simulink model "Simulink Deliverable 1"  (R2020a)
settings: Solver=FixedStepAuto  StartTime=0.0  StopTime=10.0  FixedStep=1e-3  RelTol=1e-3  EnableMultiTasking=on
undefined symbols (not defined in the file or in its folder): D0, D1, D10, D11, D12, D13, D2, D3, D4, D5, D6, D7, D8, D9, PTA0, PTA1, PTA2, PTB23, PTB9, PTC16, PTC17, PTC2, PTC3, PTC4, PTD0, PTD1, PTD2, PTD3
libraries: frdmk64flib x17
settings Model: ExtModeTrigDuration=5  Creator=shivr  LastModifiedBy=22538
settings OptimizationCC: EnhancedBackFolding=on  PassReuseOutputArgsAs=Individual arguments  ZeroExternalMemoryAtStartup=off  ZeroInternalMemoryAtStartup=off  MaxStackSize=64  OptimizeBlockOrder=speed  DifferentSizesBufferReuse=on  OptimizationCustomize=off  EfficientTunableParamExpr=on
settings DebuggingCC: ParameterTunabilityLossMsg=error
settings HardwareCC: ProdBitPerPointer=32  ProdBitPerSizeT=32  ProdBitPerPtrDiffT=32  ProdLargestAtomicInteger=Long  ProdLargestAtomicFloat=Double  ProdWordSize=32  ProdHWDeviceType=ARM Compatible->ARM Cortex
settings SFSimCC: MATLABDynamicMemAlloc=off
settings RTWCC: SystemTargetFile=ert.tlc  HardwareBoard=NXP FRDM-K64F  TemplateMakefile=ert_default_tmf  Toolchain=GNU Tools for ARM Embedded Processors
settings CodeAppCC: ForceParamTrailComments=on  IgnoreCustomStorageClasses=off  OperatorAnnotations=on  SimulinkDataObjDesc=on  SFDataObjDesc=on  InsertBlockDesc=on

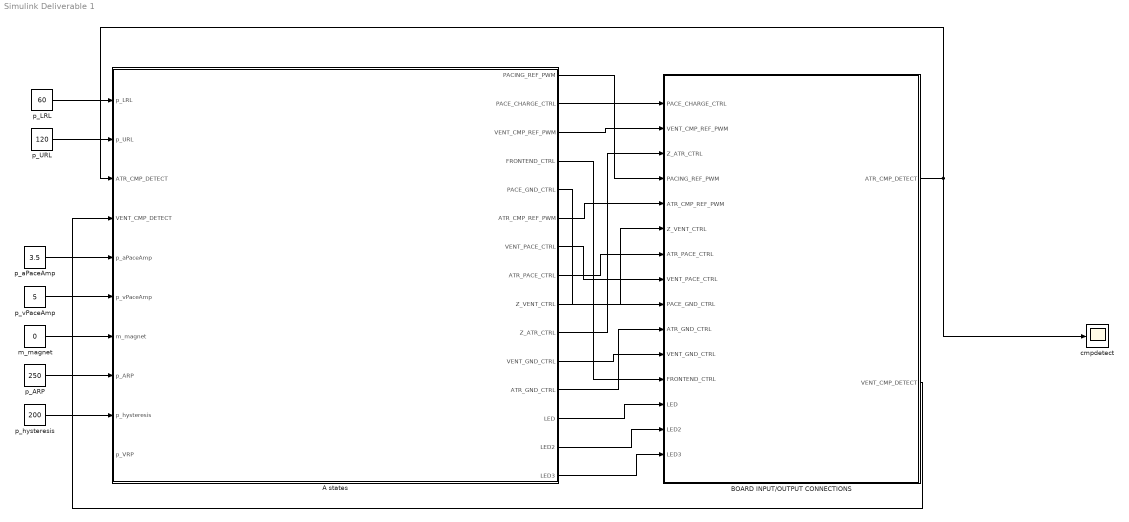
== system Simulink Deliverable 1 ==
  A states : Subsystem
  BOARD INPUT/OUTPUT CONNECTIONS : Subsystem
  cmpdetect : Scope
  m_magnet : Constant  Value=0
  p_ARP : Constant  Value=250
  p_LRL : Constant  Value=60
  p_URL : Constant  Value=120
  p_aPaceAmp : Constant  Value=3.5
  p_hysteresis : Constant  Value=200
  p_vPaceAmp : Constant  Value=5
  wires:
  p_LRL/1 -> A states/1(p_LRL)
  A states/12(ATR_GND_CTRL) -> BOARD INPUT/OUTPUT CONNECTIONS/10(ATR_GND_CTRL)
  A states/5(PACE_GND_CTRL) -> BOARD INPUT/OUTPUT CONNECTIONS/9(PACE_GND_CTRL)
  A states/11(VENT_GND_CTRL) -> BOARD INPUT/OUTPUT CONNECTIONS/11(VENT_GND_CTRL)
  A states/7(VENT_PACE_CTRL) -> BOARD INPUT/OUTPUT CONNECTIONS/8(VENT_PACE_CTRL)
  A states/8(ATR_PACE_CTRL) -> BOARD INPUT/OUTPUT CONNECTIONS/7(ATR_PACE_CTRL)
  A states/9(Z_VENT_CTRL) -> BOARD INPUT/OUTPUT CONNECTIONS/6(Z_VENT_CTRL)
  A states/10(Z_ATR_CTRL) -> BOARD INPUT/OUTPUT CONNECTIONS/3(Z_ATR_CTRL)
  A states/4(FRONTEND_CTRL) -> BOARD INPUT/OUTPUT CONNECTIONS/12(FRONTEND_CTRL)
  A states/2(PACE_CHARGE_CTRL) -> BOARD INPUT/OUTPUT CONNECTIONS/1(PACE_CHARGE_CTRL)
  A states/1(PACING_REF_PWM) -> BOARD INPUT/OUTPUT CONNECTIONS/4(PACING_REF_PWM)
  A states/13(LED) -> BOARD INPUT/OUTPUT CONNECTIONS/13(LED)
  p_URL/1 -> A states/2(p_URL)
  BOARD INPUT/OUTPUT CONNECTIONS/1(ATR_CMP_DETECT) -> A states/3(ATR_CMP_DETECT), cmpdetect/1
  BOARD INPUT/OUTPUT CONNECTIONS/2(VENT_CMP_DETECT) -> A states/4(VENT_CMP_DETECT)
  p_aPaceAmp/1 -> A states/5(p_aPaceAmp)
  m_magnet/1 -> A states/7(m_magnet)
  A states/14(LED2) -> BOARD INPUT/OUTPUT CONNECTIONS/14(LED2)
  p_vPaceAmp/1 -> A states/6(p_vPaceAmp)
  A states/6(ATR_CMP_REF_PWM) -> BOARD INPUT/OUTPUT CONNECTIONS/5(ATR_CMP_REF_PWM)
  p_ARP/1 -> A states/8(p_ARP)
  p_hysteresis/1 -> A states/9(p_hysteresis)
  A states/15(LED3) -> BOARD INPUT/OUTPUT CONNECTIONS/15(LED3)
  A states/3(VENT_CMP_REF_PWM) -> BOARD INPUT/OUTPUT CONNECTIONS/2(VENT_CMP_REF_PWM)

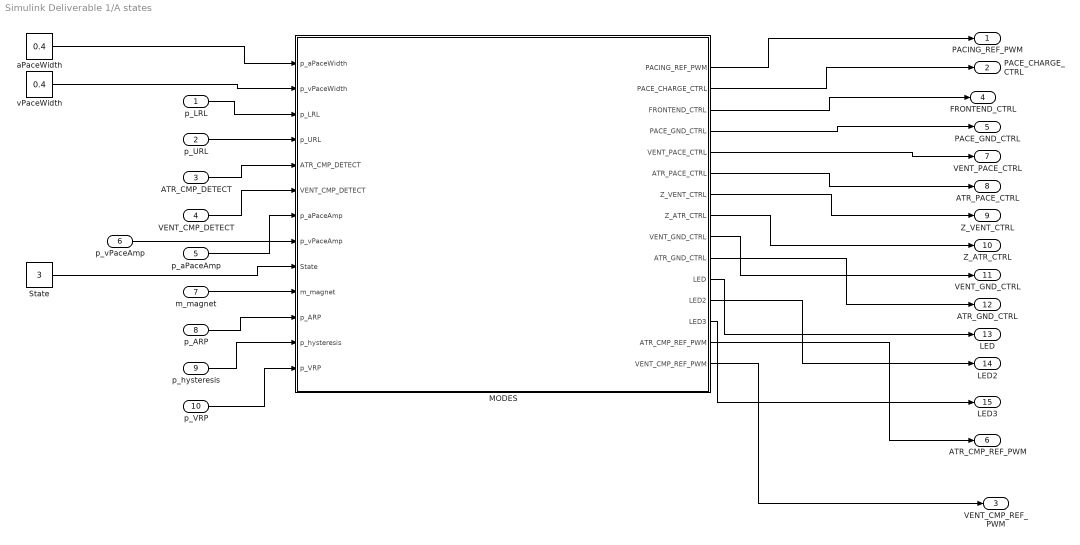
== system Simulink Deliverable 1/A states ==
  p_LRL : Inport
  p_URL : Inport  Port=2
  ATR_CMP_DETECT : Inport  Port=3
  VENT_CMP_DETECT : Inport  Port=4
  p_aPaceAmp : Inport  Port=5
  p_vPaceAmp : Inport  Port=6
  m_magnet : Inport  Port=7
  p_ARP : Inport  Port=8
  p_hysteresis : Inport  Port=9
  p_VRP : Inport  Port=10
  MODES : Stateflow chart  TreatAsAtomicUnit=on
      settings: PortSchema="{\"entries\":[{\"content\":{\"sides\":[{\"content\":{\"connectorIds\":[\"In1\",\"In2\",\"In3\",\"In4\",\"In5\",\"In6\",\"In7\",\"In8\",\"In9\",\"In10\",\"In11\",\"In12\",\"In13\"]},\"type\":\"ConnectorPlacement.EquallySpacedRectSide\",\"uuid\":\"8502a3c5-6307-4e02-81ee-17e1a35cc298\"},{\"content\":{\"connectorIds\":[\"Out1\",\"Out2\",\"Out3\",\"Out4\",\"Out5\",\"Out6\",\"Out7\",\"Out8\",\"Out9\",\"Out10\",\"Out11\",\"Out14\",\"Out13\",\"Out12\",\"Out15\"],\"side\":\"RIGHT\"},\"type\":\"ConnectorPlacement.EquallySpacedRectSide\",\"uuid\":\"71555ad9-e88e-4949-94fd-af1b739ca2ca\"},{\"content\":{\"connectorIds\":[],\"side\":\"TOP\"},\"type\":\"ConnectorPlacement.EquallySpacedRectSide\",\"uuid\":\"f0239cae-2fc2-4d44-ac00-93735ab3ef8c\"},{\"content\":{\"connectorIds\":[],\"side\":\"BOTTOM\"},\"type\":\"ConnectorPlacement.EquallySpacedRectSide\",\"uuid\":\"7d1612d5-a202-47d8-98e6-e2ca77499232\"}]},\"type\":\"ConnectorPlacement.EquallySpacedConnector\",\"uuid\":\"0a066545-78b2-4ddc-84c3-90461cea3699\"}],\"packageUris\":[\"http://schema.mathworks.com/mf0/Connector/19700101\"],\"version\":\"1.0\"}"
  State : Constant  Value=3
  aPaceWidth : Constant  Value=0.4
  vPaceWidth : Constant  Value=0.4
  PACING_REF_PWM : Outport
  PACE_CHARGE_CTRL : Outport  Port=2
  VENT_CMP_REF_PWM : Outport  Port=3
  FRONTEND_CTRL : Outport  Port=4
  PACE_GND_CTRL : Outport  Port=5
  ATR_CMP_REF_PWM : Outport  Port=6
  VENT_PACE_CTRL : Outport  Port=7
  ATR_PACE_CTRL : Outport  Port=8
  Z_VENT_CTRL : Outport  Port=9
  Z_ATR_CTRL : Outport  Port=10
  VENT_GND_CTRL : Outport  Port=11
  ATR_GND_CTRL : Outport  Port=12
  LED : Outport  Port=13
  LED2 : Outport  Port=14
  LED3 : Outport  Port=15
  wires:
  aPaceWidth/1 -> MODES/1(p_aPaceWidth)
  MODES/5(VENT_PACE_CTRL) -> VENT_PACE_CTRL/1
  MODES/3(FRONTEND_CTRL) -> FRONTEND_CTRL/1
  MODES/1(PACING_REF_PWM) -> PACING_REF_PWM/1
  MODES/6(ATR_PACE_CTRL) -> ATR_PACE_CTRL/1
  MODES/7(Z_VENT_CTRL) -> Z_VENT_CTRL/1
  MODES/4(PACE_GND_CTRL) -> PACE_GND_CTRL/1
  MODES/8(Z_ATR_CTRL) -> Z_ATR_CTRL/1
  MODES/2(PACE_CHARGE_CTRL) -> PACE_CHARGE_CTRL/1
  MODES/9(VENT_GND_CTRL) -> VENT_GND_CTRL/1
  MODES/10(ATR_GND_CTRL) -> ATR_GND_CTRL/1
  MODES/11(LED) -> LED/1
  p_LRL/1 -> MODES/3(p_LRL)
  p_URL/1 -> MODES/4(p_URL)
  ATR_CMP_DETECT/1 -> MODES/5(ATR_CMP_DETECT)
  VENT_CMP_DETECT/1 -> MODES/6(VENT_CMP_DETECT)
  p_aPaceAmp/1 -> MODES/7(p_aPaceAmp)
  State/1 -> MODES/9(State)
  m_magnet/1 -> MODES/10(m_magnet)
  MODES/14(LED2) -> LED2/1
  vPaceWidth/1 -> MODES/2(p_vPaceWidth)
  p_vPaceAmp/1 -> MODES/8(p_vPaceAmp)
  MODES/12(ATR_CMP_REF_PWM) -> ATR_CMP_REF_PWM/1
  p_ARP/1 -> MODES/11(p_ARP)
  p_hysteresis/1 -> MODES/12(p_hysteresis)
  MODES/13(LED3) -> LED3/1
  p_VRP/1 -> MODES/13(p_VRP)
  MODES/15(VENT_CMP_REF_PWM) -> VENT_CMP_REF_PWM/1

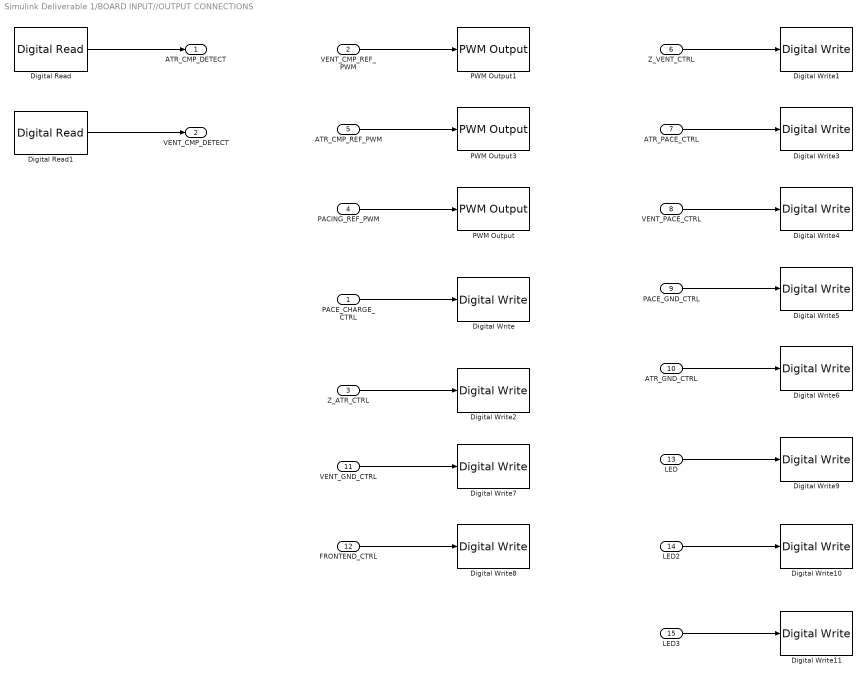
== system Simulink Deliverable 1/BOARD INPUT//OUTPUT CONNECTIONS ==
  PACE_CHARGE_CTRL : Inport
  VENT_CMP_REF_PWM : Inport  Port=2
  Z_ATR_CTRL : Inport  Port=3
  PACING_REF_PWM : Inport  Port=4
  ATR_CMP_REF_PWM : Inport  Port=5
  Z_VENT_CTRL : Inport  Port=6
  ATR_PACE_CTRL : Inport  Port=7
  VENT_PACE_CTRL : Inport  Port=8
  PACE_GND_CTRL : Inport  Port=9
  ATR_GND_CTRL : Inport  Port=10
  VENT_GND_CTRL : Inport  Port=11
  FRONTEND_CTRL : Inport  Port=12
  LED : Inport  Port=13
  LED2 : Inport  Port=14
  LED3 : Inport  Port=15
  Digital Read : frdmk64flib/Digital Read  Whichpin=PTC16 (D0)  SampleTime=-1
  Digital Read1 : frdmk64flib/Digital Read  Whichpin=PTC17 (D1)  SampleTime=-1
  Digital Write : frdmk64flib/Digital Write  Whichpin=PTB9 (D2)
  Digital Write1 : frdmk64flib/Digital Write  Whichpin=PTC3 (D7)
  Digital Write10 : frdmk64flib/Digital Write  Whichpin=BLUE_LED
  Digital Write11 : frdmk64flib/Digital Write  Whichpin=GREEN_LED
  Digital Write2 : frdmk64flib/Digital Write  Whichpin=PTB23 (D4)
  Digital Write3 : frdmk64flib/Digital Write  Whichpin=PTA0 (D8)
  Digital Write4 : frdmk64flib/Digital Write  Whichpin=PTC4 (D9)
  Digital Write5 : frdmk64flib/Digital Write  Whichpin=PTD0 (D10)
  Digital Write6 : frdmk64flib/Digital Write  Whichpin=PTD2 (D11)
  Digital Write7 : frdmk64flib/Digital Write  Whichpin=PTD3 (D12)
  Digital Write8 : frdmk64flib/Digital Write  Whichpin=PTD1 (D13)
  Digital Write9 : frdmk64flib/Digital Write  Whichpin=RED_LED
  PWM Output : frdmk64flib/PWM Output  Whichpin=PTA2 (D5)  InitialFrequency=2000  InitialDutyCycle=0
  PWM Output1 : frdmk64flib/PWM Output  Whichpin=PTA1 (D3)  InitialFrequency=2000  InitialDutyCycle=0
  PWM Output3 : frdmk64flib/PWM Output  Whichpin=PTC2 (D6)  InitialFrequency=2000  InitialDutyCycle=100
  ATR_CMP_DETECT : Outport
  VENT_CMP_DETECT : Outport  Port=2
  wires:
  Digital Read/1 -> ATR_CMP_DETECT/1
  Digital Read1/1 -> VENT_CMP_DETECT/1
  VENT_CMP_REF_PWM/1 -> PWM Output1/1
  PACE_CHARGE_CTRL/1 -> Digital Write/1
  Z_ATR_CTRL/1 -> Digital Write2/1
  PACING_REF_PWM/1 -> PWM Output/1
  ATR_CMP_REF_PWM/1 -> PWM Output3/1
  Z_VENT_CTRL/1 -> Digital Write1/1
  ATR_PACE_CTRL/1 -> Digital Write3/1
  VENT_PACE_CTRL/1 -> Digital Write4/1
  PACE_GND_CTRL/1 -> Digital Write5/1
  ATR_GND_CTRL/1 -> Digital Write6/1
  VENT_GND_CTRL/1 -> Digital Write7/1
  FRONTEND_CTRL/1 -> Digital Write8/1
  LED/1 -> Digital Write9/1
  LED2/1 -> Digital Write10/1
  LED3/1 -> Digital Write11/1

== stateflow chart Simulink Deliverable 1/A states/MODES ==
  state AOO
    state Pace
      entry:
      PACE_CHARGE_CTRL = false; %stop charging
      PACE_GND_CTRL = true;
      ATR_PACE_CTRL = true;
      ATR_GND_CTRL = false;
      Z_ATR_CTRL = false;
      Z_VENT_CTRL = false;
      VENT_GND_CTRL = false;
      VENT_PACE_CTRL = false;
      LED =true;
      %add LED as well
    state Prep
      entry:
      FRONTEND_CTRL=false; %sensing off
      %start charging C22
      ATR_PACE_CTRL = false;       %1
      VENT_PACE_CTRL = false;      %2
      PACING_REF_PWM = (p_aPaceAmp/5) * 100; %3
      PACE_CHARGE_CTRL = true;  %4
      %discharge blocking (combined state)
      PACE_GND_CTRL = false; %
      Z_ATR_CTRL= false;
      Z_VENT_CTRL=false;
      %ATR_PACE_CTRL = false;
      ATR_GND_CTRL = true;
      VENT_GND_CTRL = false;
      LED = false;
    (default) -> Prep
    Prep -> Pace : [after(60000/p_LRL-p_aPaceWidth, msec)]
    Pace -> Prep : [after(p_aPaceWidth, msec)]
  state state_selector
  state VOO
    state VOO_Prep_State
      entry:
      FRONTEND_CTRL=false;
      %charging
      ATR_PACE_CTRL = false;
      VENT_PACE_CTRL=false;
      PACING_REF_PWM = (p_vPaceAmp/5)*100;
      PACE_CHARGE_CTRL=true;
      %discharging
      PACE_GND_CTRL=true; %vp = 0
      Z_ATR_CTRL = false;
      Z_VENT_CTRL=false;
      ATR_GND_CTRL = false;
      VENT_GND_CTRL=true; %c_vp=0;
      LED2 = false;
    state VOO_Pace_State
      entry:
      PACE_CHARGE_CTRL=false;
      PACE_GND_CTRL=true;
      ATR_PACE_CTRL = false;
      ATR_GND_CTRL = false;
      Z_ATR_CTRL = false;
      Z_VENT_CTRL = false;
      VENT_GND_CTRL=false;
      VENT_PACE_CTRL=true;
      LED2 = true;
    (default) -> VOO_Prep_State
    VOO_Prep_State -> VOO_Pace_State : [after(60000.0/p_LRL - p_vPaceWidth,msec)]
    VOO_Pace_State -> VOO_Prep_State : [after(p_vPaceWidth,msec)]
  state AAI
    state AAI_CHARGING_DISCHARGING
      entry:
      FRONTEND_CTRL = true; %enable sensing
      %charge
      ATR_PACE_CTRL = false;
      PACE_CHARGE_CTRL = true;
      PACE_GND_CTRL = true;
      VENT_PACE_CTRL = false;
      PACING_REF_PWM = p_aPaceAmp/5*100;
      %discharge
      ATR_GND_CTRL = true;
      VENT_PACE_CTRL = false;
      VENT_GND_CTRL = false;
      Z_ATR_CTRL = false;
      Z_VENT_CTRL = false;
      LED3 = false;
      %Double Check
      ATR_CMP_REF_PWM = p_aPaceAmp/5*100;
      %52
    state AAI_PACING
      entry:
      FRONTEND_CTRL = false; %turn off sensing
      %pace like aoo
      PACE_CHARGE_CTRL = false;
      PACE_GND_CTRL = true;
      ATR_PACE_CTRL = true;
      ATR_GND_CTRL = false;
      VENT_PACE_CTRL = false;
      VENT_GND_CTRL = false;
      Z_VENT_CTRL = false;
      Z_ATR_CTRL = false;
      LED3 = true;
    state AAI_REFRACTORY
      entry:
      FRONTEND_CTRL = true;
      %
      PACE_CHARGE_CTRL = true;
      ATR_PACE_CTRL = false;
      VENT_PACE_CTRL = false;
      %
      ATR_GND_CTRL = true;
      PACE_GND_CTRL = true;
      VENT_PACE_CTRL = false;
      VENT_GND_CTRL = false;
      Z_ATR_CTRL=false;
      Z_VENT_CTRL = false;
      LED2 = ~LED2;
    (default) -> AAI_CHARGING_DISCHARGING
    AAI_CHARGING_DISCHARGING -> AAI_PACING [order 1] : [ATR_CMP_DETECT==false&&after((60000/p_LRL-p_aPaceWidth), msec)]
    AAI_PACING -> AAI_CHARGING_DISCHARGING : [after(p_aPaceWidth, msec)]
    AAI_REFRACTORY -> AAI_PACING [order 2] : [after((60000/p_LRL + p_hysteresis),msec)]
    AAI_REFRACTORY -> AAI_REFRACTORY [order 1] : [after(p_ARP, msec) && ATR_CMP_DETECT == true]
    AAI_CHARGING_DISCHARGING -> AAI_REFRACTORY [order 2] : [after(p_ARP, msec) && ATR_CMP_DETECT == true]
  state VVI
    state VVI_SENSING
      entry:
      FRONTEND_CTRL = true; %enable sensing
      %charge
      ATR_PACE_CTRL = false;
      PACE_CHARGE_CTRL = true;
      PACE_GND_CTRL = true;
      VENT_PACE_CTRL = false;
      PACING_REF_PWM = p_vPaceAmp/5*100;
      %discharge
      ATR_GND_CTRL =false;
      VENT_GND_CTRL = true;
      Z_ATR_CTRL = false;
      Z_VENT_CTRL = false;
      LED3 = false;
      %Double Check
      VENT_CMP_REF_PWM = p_vPaceAmp/5*100;
      %52
    state VVI_PACING
      entry:
      FRONTEND_CTRL = false; %turn off sensing
      %pace like aoo
      PACE_CHARGE_CTRL = false;
      PACE_GND_CTRL = true;
      ATR_PACE_CTRL = false;
      ATR_GND_CTRL = false;
      VENT_PACE_CTRL = true;
      VENT_GND_CTRL = false;
      Z_VENT_CTRL = false;
      Z_ATR_CTRL = false;
      LED3 = true;
    state VVI_REFRACTORY
      entry:
      FRONTEND_CTRL = true;
      %
      PACE_CHARGE_CTRL = true;
      ATR_PACE_CTRL = false;
      VENT_PACE_CTRL = false;
      %
      ATR_GND_CTRL = false;
      PACE_GND_CTRL = true;
      VENT_PACE_CTRL = false;
      VENT_GND_CTRL = true;
      Z_ATR_CTRL=false;
      Z_VENT_CTRL = false;
      LED2 = ~LED2;
    (default) -> VVI_SENSING
    VVI_SENSING -> VVI_PACING [order 1] : [VENT_CMP_DETECT==false&&after((60000/p_LRL-p_vPaceWidth), msec)]
    VVI_PACING -> VVI_SENSING : [after(p_vPaceWidth, msec)]
    VVI_REFRACTORY -> VVI_PACING [order 2] : [after((60000/p_LRL + p_hysteresis),msec)]
    VVI_REFRACTORY -> VVI_REFRACTORY [order 1] : [after(p_VRP, msec) && VENT_CMP_DETECT == true]
    VVI_SENSING -> VVI_REFRACTORY [order 2] : [after(p_VRP, msec) && VENT_CMP_DETECT == true]
  state_selector -> AOO [order 1] : [State == 1&&m_magent==0]
  (default) -> state_selector
  state_selector -> VOO [order 2] : [m_magnet == 1 || State == 2]
  state_selector -> VVI [order 4] : [State == 4&&m_magnet==0]
  state_selector -> AAI [order 3] : [State == 3&&m_magnet==0]
  data: PACING_REF_PWM output; PACE_CHARGE_CTRL output; FRONTEND_CTRL output; PACE_GND_CTRL output; VENT_PACE_CTRL output; ATR_PACE_CTRL output; Z_VENT_CTRL output; Z_ATR_CTRL output; VENT_GND_CTRL output; ATR_GND_CTRL output; LED output; ATR_CMP_REF_PWM output; LED3 output; p_aPaceWidth input; p_vPaceWidth input; p_LRL input; p_URL input; ATR_CMP_DETECT input; VENT_CMP_DETECT input; p_aPaceAmp input; p_vPaceAmp input; State input; m_magnet input; LED2 output; p_ARP input; p_hysteresis input; p_VRP input; VENT_CMP_REF_PWM output
